simulink model "USCS_Soil_Model"  (R2020a)
settings: Solver=VariableStepAuto  StartTime=0.0  StopTime=10.0  RelTol=1e-3
libraries: simulink x4
settings Model: Creator=SMONE  LastModifiedBy=SMONE

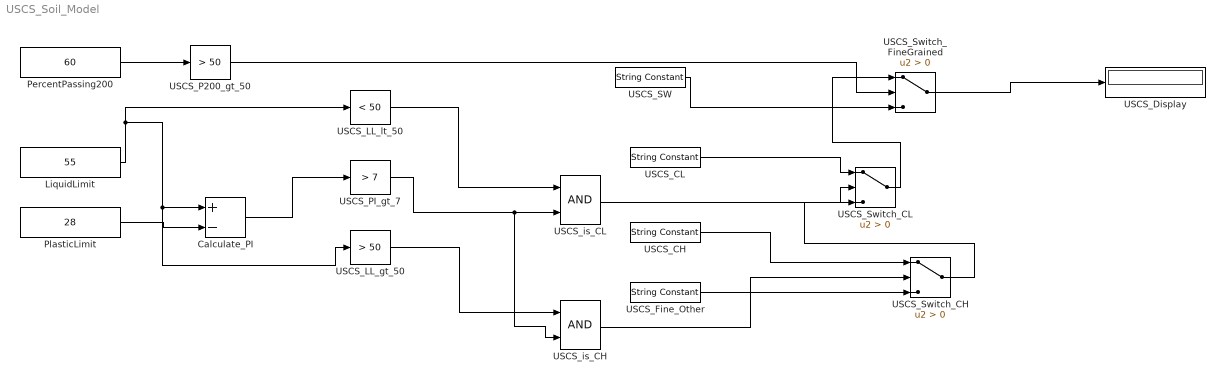
== system USCS_Soil_Model ==
  Calculate_PI : Sum  Inputs=+-
  LiquidLimit : Constant  Value=55
  PercentPassing200 : Constant  Value=60
  PlasticLimit : Constant  Value=28
  USCS_CH : StringConstant  String='CH'
  USCS_CL : StringConstant  String='CL'
  USCS_Display : Display
  USCS_Fine_Other : StringConstant  String='Fine (Other)'
  USCS_LL_gt_50 : simulink/Logic and Bit Operations/Compare To Constant  relop=>  const=50  OutDataTypeStr=boolean
  USCS_LL_lt_50 : simulink/Logic and Bit Operations/Compare To Constant  relop=<  const=50  OutDataTypeStr=boolean
  USCS_P200_gt_50 : simulink/Logic and Bit Operations/Compare To Constant  relop=>  const=50  OutDataTypeStr=boolean
  USCS_PI_gt_7 : simulink/Logic and Bit Operations/Compare To Constant  relop=>  const=7  OutDataTypeStr=boolean
  USCS_SW : StringConstant  String='SW (Coarse)'
  USCS_Switch_CH : Switch  Criteria=u2 > Threshold
  USCS_Switch_CL : Switch  Criteria=u2 > Threshold
  USCS_Switch_FineGrained : Switch  Criteria=u2 > Threshold
  USCS_is_CH : Logic  AllPortsSameDT=off  OutDataTypeStr=boolean
  USCS_is_CL : Logic  AllPortsSameDT=off  OutDataTypeStr=boolean
  wires:
  LiquidLimit/1 -> USCS_LL_gt_50/1, Calculate_PI/1, USCS_LL_lt_50/1
  PlasticLimit/1 -> Calculate_PI/2
  PercentPassing200/1 -> USCS_P200_gt_50/1
  Calculate_PI/1 -> USCS_PI_gt_7/1
  USCS_LL_lt_50/1 -> USCS_is_CL/1
  USCS_PI_gt_7/1 -> USCS_is_CH/2, USCS_is_CL/2
  USCS_LL_gt_50/1 -> USCS_is_CH/1
  USCS_Fine_Other/1 -> USCS_Switch_CH/3
  USCS_CH/1 -> USCS_Switch_CH/1
  USCS_is_CH/1 -> USCS_Switch_CH/2
  USCS_Switch_CH/1 -> USCS_Switch_CL/3
  USCS_CL/1 -> USCS_Switch_CL/1
  USCS_is_CL/1 -> USCS_Switch_CL/2
  USCS_Switch_CL/1 -> USCS_Switch_FineGrained/1
  USCS_SW/1 -> USCS_Switch_FineGrained/3
  USCS_P200_gt_50/1 -> USCS_Switch_FineGrained/2
  USCS_Switch_FineGrained/1 -> USCS_Display/1
